simulink model "Final_System_Model_V2"  (R2018a)
settings: Solver=VariableStepAuto  StartTime=0  StopTime=inf  RelTol=1e-3
PreLoadFcn:
  | Ts_Power=1e-6;
  | Ts_Control=100e-6;
undefined symbols (not defined in the file): DiscIntNeverNeededParam, FC, FuelCellLoadFcn, gcbh, Ion, Lithium, sigbuilder_block, sps_rtmsupport
libraries: powerlib x20, simulink x10, fl_lib x8, nesl_utility x6, powerlib_meascontrol x5, electricdrivelib x1, spsFuelCellModel x1, re_lib x1
(part 4 of 4)

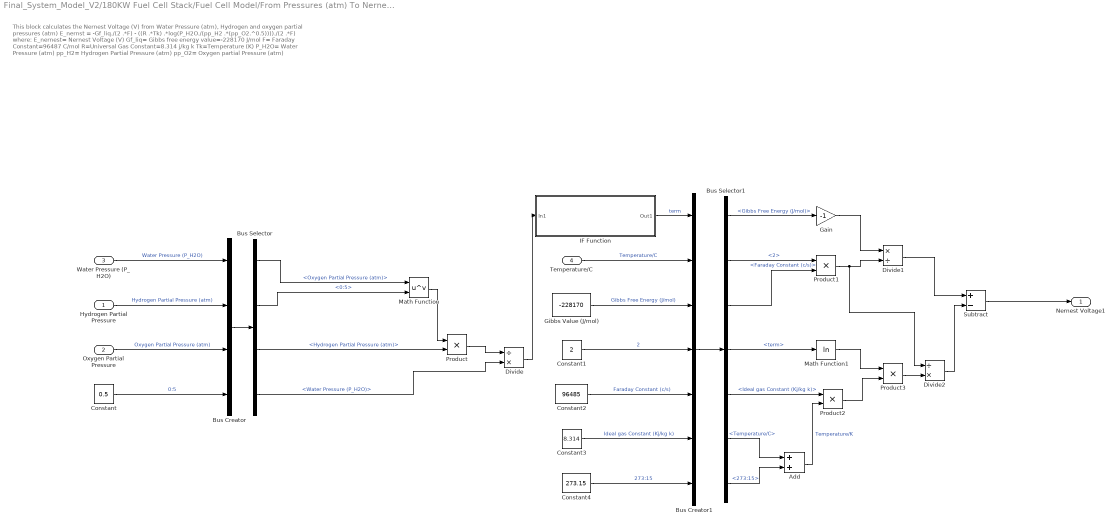
== system Final_System_Model_V2/180KW Fuel Cell Stack/Fuel Cell Model/From Pressures (atm) To Nernest Voltage (V)/From Partial Pressures (atm) To Nernest Voltage (V) ==
  note: This block calculates the Nernest Voltage (V) from Water Pressure (atm), Hydrogen and oxygen partial pressures (atm)
      | E_nernst = -Gf_liq./(2 .*F) - ((R .*Tk) .*log(P_H2O./(pp_H2 .*(pp_O2.^0.5))))./(2 .*F)
      | where: E_nernest= Nernest Voltage (V)
      | Gf_liq= Gibbs free energy value=-228170 J/mol
      | F= Faraday Constant=96487 C/mol
      | R=Universal Gas Constant=8.314 j/kg k
      | Tk=Temperature (K)
      | P_H2O= Water Pressure (atm)
      | pp_H2= Hydrogen Partial Pressure (atm)
      | pp_O2= Oxygen partial Pressure (atm)
  Hydrogen Partial Pressure : Inport
  Oxygen Partial Pressure : Inport  Port=2
  Water Pressure (P_H2O) : Inport  Port=3
  Temperature/C : Inport  Port=4
  Add : Sum
  Bus Creator : BusCreator  Inputs=4
  Bus Creator1 : BusCreator  Inputs=7
  Bus Selector : BusSelector  OutputSignals=Oxygen Partial Pressure (atm),0:5,Hydrogen Partial Pressure (atm),Water Pressure (P_H2O)
  Bus Selector1 : BusSelector  OutputSignals=Gibbs Free Energy (J/mol),2,Faraday Constant (c/s),term,Ideal gas Constant (Kj/kg k),Temperature/C,273:15
  Constant : Constant  Value=0.5
  Constant1 : Constant  Value=2
  Constant2 : Constant  Value=96485
  Constant3 : Constant  Value=8.314
  Constant4 : Constant  Value=273.15
  Divide : Product  Inputs=/*
  Divide1 : Product  Inputs=*/
  Divide2 : Product  Inputs=/*
  Gain : Gain  Gain=-1
  Gibbs Value (J/mol) : Constant  Value=-228170
  IF Function : Subsystem
  Math Function : Math  Operator=pow  SaturateOnIntegerOverflow=on
  Math Function1 : Math  Operator=log  SaturateOnIntegerOverflow=on
  Product{,1..3} (4 alike) : Product
  Subtract : Sum  Inputs=+-
  Nernest Voltage1 : Outport
  wires:
  Gibbs Value (J/mol)/1 -> Bus Creator1/3  "Gibbs Free Energy (J/mol)"
  Oxygen Partial Pressure/1 -> Bus Creator/3  "Oxygen Partial Pressure (atm)"
  Water Pressure (P_H2O)/1 -> Bus Creator/1  "Water Pressure (P_H2O)"
  Hydrogen Partial Pressure/1 -> Bus Creator/2  "Hydrogen Partial Pressure (atm)"
  Temperature/C/1 -> Bus Creator1/2  "Temperature/C"
  Bus Creator/1 -> Bus Selector/1
  Bus Selector/2 -> Math Function/2  "<0:5>"
  Constant/1 -> Bus Creator/4  "0:5"
  Bus Selector/1 -> Math Function/1  "<Oxygen Partial Pressure (atm)>"
  Bus Selector/3 -> Product/2  "<Hydrogen Partial Pressure (atm)>"
  Math Function/1 -> Product/1
  Bus Selector/4 -> Divide/2  "<Water Pressure (P_H2O)>"
  Product/1 -> Divide/1
  Divide/1 -> IF Function/1(In1)
  IF Function/1(Out1) -> Bus Creator1/1  "term"
  Bus Creator1/1 -> Bus Selector1/1
  Constant1/1 -> Bus Creator1/4  "2"
  Constant2/1 -> Bus Creator1/5  "Faraday Constant (c/s)"
  Bus Selector1/1 -> Gain/1  "<Gibbs Free Energy (J/mol)>"
  Gain/1 -> Divide1/1
  Bus Selector1/2 -> Product1/1  "<2>"
  Bus Selector1/3 -> Product1/2  "<Faraday Constant (c/s)>"
  Product1/1 -> Divide2/1, Divide1/2
  Divide1/1 -> Subtract/1
  Bus Selector1/4 -> Math Function1/1  "<term>"
  Math Function1/1 -> Product3/1
  Constant3/1 -> Bus Creator1/6  "Ideal gas Constant (Kj/kg k)"
  Constant4/1 -> Bus Creator1/7  "273:15"
  Bus Selector1/5 -> Product2/1  "<Ideal gas Constant (Kj/kg k)>"
  Bus Selector1/6 -> Add/1  "<Temperature/C>"
  Bus Selector1/7 -> Add/2  "<273:15>"
  Add/1 -> Product2/2  "Temperature/K"
  Product2/1 -> Product3/2
  Product3/1 -> Divide2/2
  Divide2/1 -> Subtract/2
  Subtract/1 -> Nernest Voltage1/1

== system Final_System_Model_V2/Electrolyzer Stack/electrolyser stack/electrolyser cell/(1//T)//(1//T_ref) ==
  In1 : Inport
  In2 : Inport  Port=2
  Constant : Constant
  Divide1 : Product  Inputs=*/
  Divide2 : Product  Inputs=*/
  Out1 : Outport
  wires:
  Divide1/1 -> Divide2/1
  Constant/1 -> Divide1/1
  In2/1 -> Divide2/2
  Divide2/1 -> Out1/1
  In1/1 -> Divide1/2

== system Final_System_Model_V2/Electrolyzer Stack/electrolyser stack/electrolyser cell/Eta_B ==
  In1 : Inport
  In2 : Inport  Port=2
  In3 : Inport  Port=3
  In4 : Inport  Port=4
  L_B : Constant  Value=175e-4
  Product : Product  Inputs=*/
  Product1 : Product
  segma_B : Subsystem
  Out1 : Outport
  wires:
  segma_B/1(Out1) -> Product/2
  L_B/1 -> Product/1
  Product1/1 -> Out1/1
  In3/1 -> Product1/2
  Product/1 -> Product1/1
  In2/1 -> segma_B/2(In2)
  In4/1 -> segma_B/3(In4)
  In1/1 -> segma_B/1(In1)

== system Final_System_Model_V2/Electrolyzer Stack/electrolyser stack/electrolyser cell/H2 flow rate ==
  In1 : Inport
  In2 : Inport  Port=2
  In3 : Inport  Port=3
  Divide : Product  Inputs=*/
  Multiply : Product
  Out1 : Outport
  wires:
  Multiply/1 -> Divide/1
  In1/1 -> Multiply/1
  In3/1 -> Multiply/2
  In2/1 -> Divide/2
  Divide/1 -> Out1/1

== system Final_System_Model_V2/Electrolyzer Stack/electrolyser stack/electrolyser cell/V_0 ==
  In1 : Inport
  Add : Sum  Inputs=+-
  Add1 : Sum  Inputs=+-
  Constant : Constant  Value=8.46e-4
  OCV : Constant  Value=1.229
  Product : Product
  T_ref : Constant  Value=298
  Out1 : Outport
  wires:
  OCV/1 -> Add/1
  Add/1 -> Out1/1
  Product/1 -> Add/2
  T_ref/1 -> Add1/2
  In1/1 -> Add1/1
  Constant/1 -> Product/1
  Add1/1 -> Product/2

== system Final_System_Model_V2/Electrolyzer Stack/electrolyser stack/electrolyser cell/eta_a ==
  In1 : Inport
  In2 : Inport  Port=2
  In3 : Inport  Port=3
  In4 : Inport  Port=4
  In5 : Inport  Port=5
  In6 : Inport  Port=6
  B_a : Constant  Value=5
  Divide : Product  Inputs=*/
  Divide1 : Product  Inputs=*/
  Gain : Gain  Gain=0.5
  Multiply : Product
  Multiply1 : Product  Inputs=3
  Multiply2 : Product
  Sin : Trigonometry  Operator=asinh
  m_a : Subsystem
  n_a : Subsystem
  v_a : Constant  Value=3
  Out1 : Outport
  wires:
  n_a/1(Out1) -> Divide1/1
  B_a/1 -> Multiply1/1
  Divide1/1 -> Gain/1
  In1/1 -> n_a/1(In1)
  Sin/1 -> Multiply2/1
  Multiply/1 -> Divide/1
  In6/1 -> Multiply1/3
  Gain/1 -> Sin/1
  Multiply1/1 -> Divide/2
  In3/1 -> n_a/3(In3), m_a/1(In1)
  Multiply2/1 -> Out1/1
  Divide/1 -> Multiply2/2
  v_a/1 -> Multiply1/2
  m_a/1(Out1) -> Divide1/2
  In5/1 -> Multiply/2
  In4/1 -> Multiply/1
  In2/1 -> n_a/2(In2)

== system Final_System_Model_V2/Electrolyzer Stack/electrolyser stack/electrolyser cell/eta_c ==
  In1 : Inport
  In2 : Inport  Port=2
  In3 : Inport  Port=3
  In4 : Inport  Port=4
  In5 : Inport  Port=5
  B_c : Constant  Value=5
  Divide : Product  Inputs=*/
  Divide1 : Product  Inputs=*/
  Gain : Gain  Gain=0.5
  Multiply : Product
  Multiply1 : Product  Inputs=3
  Multiply2 : Product
  Sin : Trigonometry  Operator=asinh
  m_c : Subsystem
  n_c : Subsystem
  v_c : Constant  Value=-1
  Out1 : Outport
  wires:
  In1/1 -> n_c/1(In1)
  In2/1 -> Multiply/1, n_c/2(In2)
  Multiply/1 -> Divide/1
  Divide1/1 -> Gain/1
  n_c/1(Out1) -> Divide1/1
  v_c/1 -> Multiply1/3
  In4/1 -> m_c/1(In1), n_c/3(In3)
  B_c/1 -> Multiply1/1
  Multiply1/1 -> Divide/2
  Sin/1 -> Multiply2/1
  m_c/1(Out1) -> Divide1/2
  Divide/1 -> Multiply2/2
  Gain/1 -> Sin/1
  Multiply2/1 -> Out1/1
  In3/1 -> Multiply/2
  In5/1 -> Multiply1/2

== system Final_System_Model_V2/Solar Panel + Solar Charge Controller/PV Insert inputs here/Subsystem/C to K Converter  ==
  T_o : Inport
  Sum : Sum  Inputs=|++
  Sum1 : Sum  Inputs=|++
  T_ref : Constant  Value=25
  constant : Constant  Value=273.12
  T_ak : Outport
  T_rk : Outport  Port=2
  wires:
  constant/1 -> Sum1/1, Sum/2
  T_o/1 -> Sum/1  "T_act (c)"
  T_ref/1 -> Sum1/2  "T_ref (c)"
  Sum/1 -> T_ak/1  "T_act(k)"
  Sum1/1 -> T_rk/1  "T_ref(k)"

== system Final_System_Model_V2/Solar Panel + Solar Charge Controller/PV Insert inputs here/Subsystem/I o ==
  T_ak : Inport
  T_rk : Inport  Port=2
  I_on : Inport  Port=3
  Constant : Constant
  Electron charge : Constant  Value=1.6*10^(-19)
  Exp(fn(1)) : Fcn  Expr=exp(u(1))
  Fcn : Fcn  Expr=(u(1))^3
  Product : Product  Inputs=/***/
  Product1 : Product  Inputs=*/
  Product2 : Product  Inputs=*/
  Product3 : Product  Inputs=*/
  Product4 : Product  Inputs=3
  Sum : Sum  Inputs=|+-
  band gap energy (Eg) : Constant  Value=1.1
  boltzamann constant : Constant  Value=1.3805*10^(-23)
  ideality factor depend on material : Constant  Value=1.14
  I_o : Outport
  wires:
  Electron charge/1 -> Product/2  "e"
  boltzamann constant/1 -> Product/1  "k"
  Product2/1 -> Sum/2  "1/T"
  I_on/1 -> Product4/3  "I_on"
  band gap energy (Eg)/1 -> Product/3  "Eg"
  Sum/1 -> Product/4  "((1/Tn)-(1/T))"
  Product3/1 -> Fcn/1  "T/Tn"
  Product1/1 -> Sum/1  "1/Tn"
  Constant/1 -> Product2/1, Product1/1
  ideality factor depend on material/1 -> Product/5  "a"
  T_ak/1 -> Product3/1, Product2/2
  Fcn/1 -> Product4/2  "(T/Tn)^3"
  Product/1 -> Exp(fn(1))/1  "Fn(1)"
  Exp(fn(1))/1 -> Product4/1  "Exp(fn(1))"
  T_rk/1 -> Product1/2, Product3/2
  Product4/1 -> I_o/1

== system Final_System_Model_V2/Solar Panel + Solar Charge Controller/PV Insert inputs here/Subsystem/I on ==
  T_ref : Inport
  I_scn : Inport  Port=2
  Num series : Inport  Port=3
  V_oc : Inport  Port=4
  Electron charge : Constant  Value=1.6*10^(-19)
  Fcn : Fcn  Expr=(u(1))/(exp(u(2))-u(1))
  Mux : Mux  Inputs=3
  Product : Product  Inputs=//**//
  boltzamann constant : Constant  Value=1.3805*10^(-23)
  constant : Constant
  ideality factor : Constant  Value=1.1415
  I_on : Outport
  wires:
  Num series/1 -> Product/1  "num_series_cells"
  boltzamann constant/1 -> Product/2  "K"
  Electron charge/1 -> Product/3  "q"
  ideality factor/1 -> Product/5  "a"
  T_ref/1 -> Product/6  "T_ref(k)"
  Product/1 -> Mux/2
  I_scn/1 -> Mux/1
  constant/1 -> Mux/3
  Mux/1 -> Fcn/1
  Fcn/1 -> I_on/1
  V_oc/1 -> Product/4

== system Final_System_Model_V2/Solar Panel + Solar Charge Controller/PV Insert inputs here/Subsystem/I ph due to radiation  ==
  insolation : Inport
  T_ak : Inport  Port=2
  T_rk : Inport  Port=3
  I_scn : Inport  Port=4
  Product : Product
  Product1 : Product
  SC_temp COFF const : Constant  Value=0.0017
  Sum : Sum  Inputs=|++
  Sum1 : Sum  Inputs=|+-
  I_photon : Outport
  wires:
  Product/1 -> I_photon/1  "photons current"
  insolation/1 -> Product/1
  T_ak/1 -> Sum1/1  "actual temp(k)"
  T_rk/1 -> Sum1/2  "referance temp(k)"
  Sum/1 -> Product/2
  I_scn/1 -> Sum/2  "nominal short circuit current"
  Product1/1 -> Sum/1
  SC_temp COFF const/1 -> Product1/1
  Sum1/1 -> Product1/2

== system Final_System_Model_V2/Solar Panel + Solar Charge Controller/PV Insert inputs here/Subsystem/I pv ==
  V_PV : Inport
  I_photon : Inport  Port=2
  I_o : Inport  Port=3
  Ns*A*Kt1 : Inport  Port=4
  Rp Shunt resistance : Inport  Port=5
  Electron charge : Constant  Value=1.6*10^(-19)
  IPV = u(3)-u(4)*(exp((u(2)*(u(1)+u(6)))/(u(5)))-1) : Fcn  Expr=u(3)-u(4)*(exp((u(2)*(u(1)+u(6)))/(u(5)))-1)-u(7)
  Mux : Mux  Inputs=7
  Product : Product  Inputs=*/
  Rs : Gain  Gain=.4
  Sum : Sum  Inputs=|++
  I_PV : Outport
  wires:
  IPV = u(3)-u(4)*(exp((u(2)*(u(1)+u(6)))/(u(5)))-1)/1 -> I_PV/1, Rs/1  "I_PV"
  Ns*A*Kt1/1 -> Mux/5
  Mux/1 -> IPV = u(3)-u(4)*(exp((u(2)*(u(1)+u(6)))/(u(5)))-1)/1
  I_o/1 -> Mux/4  "I_o"
  Rs/1 -> Sum/2, Mux/6  "I_PV*Rs"
  Electron charge/1 -> Mux/2  "q"
  I_photon/1 -> Mux/3  "I_ph"
  V_PV/1 -> Sum/1, Mux/1  "V_PV"
  Sum/1 -> Product/1
  Rp Shunt resistance/1 -> Product/2  "Shunt resistance"
  Product/1 -> Mux/7

== system Final_System_Model_V2/Solar Panel + Solar Charge Controller/PV Insert inputs here/Subsystem/NsAKt Thermal voltafe ==
  T_ak T in kelven : Inport
  N_series series cells : Constant  Value=96
  Product4 : Product  Inputs=4
  boltzamann constant : Constant  Value=1.3805*10^(-23)
  ideality factor depend on material : Constant  Value=1.17
  Ns*a*Kt : Outport
  wires:
  Product4/1 -> Ns*a*Kt/1
  boltzamann constant/1 -> Product4/2
  ideality factor depend on material/1 -> Product4/3
  T_ak T in kelven/1 -> Product4/1
  N_series series cells/1 -> Product4/4

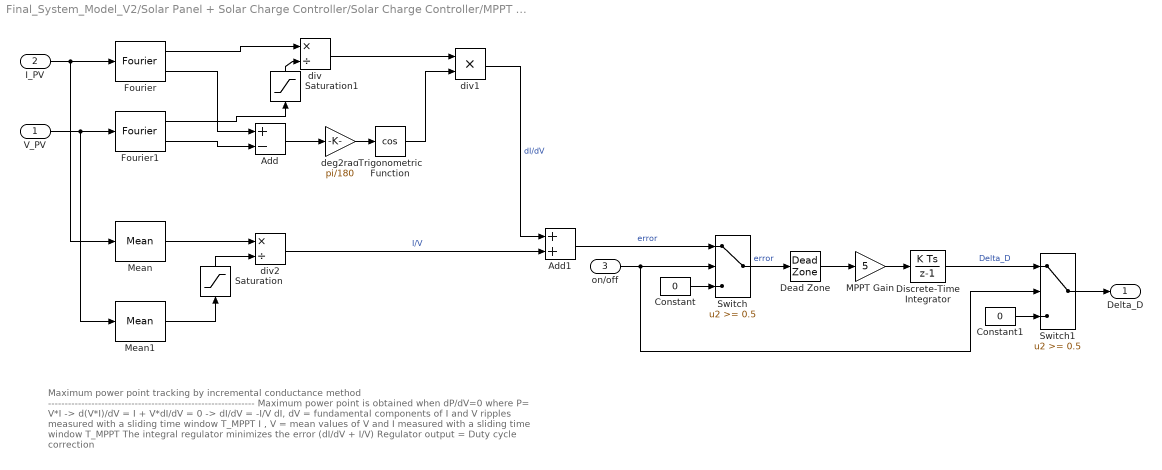
== system Final_System_Model_V2/Solar Panel + Solar Charge Controller/Solar Charge Controller/MPPT Controller using  "Incremental Conductance + Integral Regulator "  technique /MPPT ==
  note: Maximum power point tracking by incremental conductance method
      | --------------------------------------------------------------
      | Maximum power point is obtained when dP/dV=0  where P= V*I
      | -> d(V*I)/dV = I + V*dI/dV = 0
      | -> dI/dV = -I/V
      |
      | dI, dV  = fundamental components of I and V ripples measured with a sliding time window T_MPPT
      | I , V   = mean values of V and I measured with a sliding time window T_MPPT
      |
      | The integral regulator minimizes the error (dI/dV + I/V)
      | Regulator output = Duty cycle correction
  V_PV : Inport
  I_PV : Inport  Port=2
  on/off : Inport  Port=3
  Add : Sum  Inputs=+-
  Add1 : Sum
  Constant : Constant  Value=0
  Constant1 : Constant  Value=0
  Dead Zone : DeadZone  LowerValue=-0.05  UpperValue=0.05  SaturateOnIntegerOverflow=on
  Discrete-Time Integrator : DiscreteIntegrator  SampleTime=Ts_Control  LimitOutput=on  UpperSaturationLimit=1  LowerSaturationLimit=-1  ICPrevOutput=DiscIntNeverNeededParam  ICPrevScaledInput=DiscIntNeverNeededParam
  Fourier : powerlib_meascontrol/Measurements/Fourier  Freq=1/T_MPPT  n=1  InInit=[0, 0]  Ts=Ts_Control
      settings: SourceProductName=Simscape Power Systems
  Fourier1 : powerlib_meascontrol/Measurements/Fourier  Freq=1/T_MPPT  n=1  InInit=[0, 0]  Ts=Ts_Control
      settings: SourceProductName=Simscape Power Systems
  MPPT Gain : Gain  Gain=5
  Mean : powerlib_meascontrol/Measurements/Mean  Freq=1/T_MPPT  Vinit=0  Ts=Ts_Control
  Mean1 : powerlib_meascontrol/Measurements/Mean  Freq=1/T_MPPT  Vinit=0  Ts=Ts_Control
  Saturation : Saturate  UpperLimit=inf  LowerLimit=eps
  Saturation1 : Saturate  UpperLimit=inf  LowerLimit=eps
  Switch : Switch  Threshold=0.5
  Switch1 : Switch  Threshold=0.5
  Trigonometric Function : Trigonometry  Operator=cos
  deg2rad : Gain  Gain=pi/180
  div : Product  Inputs=*/  RndMeth=Zero
  div1 : Product  Inputs=**  RndMeth=Zero
  div2 : Product  Inputs=*/  RndMeth=Zero
  Delta_D : Outport
  wires:
  Dead Zone/1 -> MPPT Gain/1
  Switch/1 -> Dead Zone/1  "error"
  Saturation1/1 -> div/2
  Saturation/1 -> div2/2
  Switch1/1 -> Delta_D/1
  on/off/1 -> Switch/2, Switch1/2
  Constant1/1 -> Switch1/3
  Discrete-Time Integrator/1 -> Switch1/1  "Delta_D"
  Constant/1 -> Switch/3
  MPPT Gain/1 -> Discrete-Time Integrator/1
  Add1/1 -> Switch/1  "error"
  div2/1 -> Add1/2  "I/V"
  Mean1/1 -> Saturation/1
  Mean/1 -> div2/1
  div1/1 -> Add1/1  "dI/dV"
  Trigonometric Function/1 -> div1/2
  div/1 -> div1/1
  deg2rad/1 -> Trigonometric Function/1
  Add/1 -> deg2rad/1
  Fourier1/1 -> Saturation1/1
  Fourier1/2 -> Add/2
  Fourier/2 -> Add/1
  V_PV/1 -> Mean1/1, Fourier1/1
  I_PV/1 -> Mean/1, Fourier/1
  Fourier/1 -> div/1

== system Final_System_Model_V2/Solar Panel + Solar Charge Controller/Solar Charge Controller MPPT it is a device which track a point which has the max power/MPPT /P&O  ==
  I_pv : Inport
  V_PV : Inport  Port=2
  P & O : Subsystem
  Saturation : Saturate  UpperLimit=1
  Subsystem1 : Subsystem
  Signal : Outport
  wires:
  P & O/1(signal) -> Saturation/1
  V_PV/1 -> P & O/2(Vpv)
  Saturation/1 -> Subsystem1/1(In1)
  Subsystem1/1(Out1) -> Signal/1
  I_pv/1 -> P & O/1(Ipv)

== system Final_System_Model_V2/180KW Fuel Cell Stack/Fuel Cell Model/ From Current Density (A//cm^2) To Overvoltages (V)/Concentration Overvoltage/IF Function ==
  In1 : Inport
  Compare To Zero : simulink/Logic and Bit Operations/Compare To Zero  relop=<=  OutDataTypeStr=boolean
  If : If  IfExpression=u1 == 0
  If Action Subsystem : Subsystem  TreatAsAtomicUnit=on
  If Action Subsystem1 : Subsystem  TreatAsAtomicUnit=on
  Merge : Merge  InitialOutput=1
  Out1 : Outport
  wires:
  If Action Subsystem1/1(Out1) -> Merge/2
  Compare To Zero/1 -> If/1
  Merge/1 -> Out1/1
  In1/1 -> If Action Subsystem/1(In1), Compare To Zero/1
  If/2 -> If Action Subsystem1/Action
  If Action Subsystem/1(Out1) -> Merge/1
  If/1 -> If Action Subsystem/Action

== system Final_System_Model_V2/180KW Fuel Cell Stack/Fuel Cell Model/From Pressures (atm) To Nernest Voltage (V)/From Absolute Pressure (atm) To Partial Pressures (atm)/Hydrogen Partial Pressure Output ==
  note: This block calculates the Hydrogen partial Pressure (pp_H2)(atm)
      | pp_H2 = 0.5 .*((P_H2)./(exp(1.653 .*i./(Tk.^1.334))))-P_H2O
      | where: pp_H2= Hydrogen Partial Pressure (atm)
      | i=Current Density (A/cm^2)
      | Tk= Temperature in Kelvin
      | P_H2O= Water pressure (atm)
  Hydrogen Pressure (P_H2) : Inport
  Temperature/C : Inport  Port=2
  Current Density (i ) : Inport  Port=3
  Water Pressure : Inport  Port=4
  Add : Sum
  Bus Creator : BusCreator  Inputs=6
  Bus Selector : BusSelector  OutputSignals=Stack Temperature (C),273:15,1:653,Current Density (A/cm^2),Hydrogen Pressure (atm),Water Pressure(atm)
  Constant : Constant  Value=273.15
  Constant1 : Constant  Value=1.653
  Constant2 : Constant  Value=1.334
  Divide : Product  Inputs=/*
  Divide1 : Product  Inputs=/*
  Gain : Gain  Gain=0.5
  Math Function : Math  Operator=pow  SaturateOnIntegerOverflow=on
  Math Function1 : Math  SaturateOnIntegerOverflow=on
  Product : Product
  Subtract : Sum  Inputs=+-
  Hydrogen Partial Pressure (pp_H2) : Outport
  wires:
  Water Pressure/1 -> Bus Creator/4
  Temperature/C/1 -> Bus Creator/3
  Current Density (i )/1 -> Bus Creator/2
  Hydrogen Pressure (P_H2)/1 -> Bus Creator/1
  Bus Creator/1 -> Bus Selector/1
  Bus Selector/5 -> Divide1/2  "<Hydrogen Pressure (atm)>"
  Bus Selector/1 -> Add/1  "<Stack Temperature (C)>"
  Constant/1 -> Bus Creator/5  "273:15"
  Add/1 -> Math Function/1  "Temperature/K"
  Constant1/1 -> Bus Creator/6  "1:653"
  Bus Selector/2 -> Add/2  "<273:15>"
  Bus Selector/3 -> Product/1  "<1:653>"
  Bus Selector/4 -> Product/2  "<Current Density (A/cm^2)>"
  Product/1 -> Divide/2
  Divide/1 -> Math Function1/1
  Constant2/1 -> Math Function/2
  Math Function/1 -> Divide/1
  Math Function1/1 -> Divide1/1
  Divide1/1 -> Gain/1
  Bus Selector/6 -> Subtract/2  "<Water Pressure(atm)>"
  Subtract/1 -> Hydrogen Partial Pressure (pp_H2)/1
  Gain/1 -> Subtract/1

== system Final_System_Model_V2/180KW Fuel Cell Stack/Fuel Cell Model/From Pressures (atm) To Nernest Voltage (V)/From Absolute Pressure (atm) To Partial Pressures (atm)/Oxygen Partial Pressure Output ==
  note: This block calculates the Oxygen Partial Pressure (atm)
      | pp_O2 = (P_air./exp(4.192 .*i/(Tk.^1.334)))-P_H2O
      |
      | where: pp_O2= Oxygen Partial Pressure (atm)
      | P_air= Air Pressure (atm)
      | i= Current Density (A/cm^2)
      | Tk= Temperature (K)
      | P_H2O=Water Pressure (atm)
  Air Pressure (P_air) : Inport
  Temperature/C : Inport  Port=2
  Current Density/i : Inport  Port=3
  Water Pressure : Inport  Port=4
  Add : Sum
  Bus Creator : BusCreator  Inputs=7
  Bus Selector : BusSelector  OutputSignals=Stack Temperature (C),273:15,1:334,Current Density (A/cm^2),4:192,Air Pressure (atm),Water Pressure(atm)
  Constant : Constant  Value=273.15
  Constant1 : Constant  Value=4.192
  Constant2 : Constant  Value=1.334
  Divide : Product  Inputs=/*
  Divide1 : Product  Inputs=/*
  Math Function : Math  Operator=pow  SaturateOnIntegerOverflow=on
  Math Function1 : Math  SaturateOnIntegerOverflow=on
  Product : Product
  Subtract : Sum  Inputs=+-
  Oxygen Partial Pressure pp_O2 : Outport
  wires:
  Current Density/i/1 -> Bus Creator/2
  Water Pressure/1 -> Bus Creator/4
  Temperature/C/1 -> Bus Creator/3
  Air Pressure (P_air)/1 -> Bus Creator/1
  Constant/1 -> Bus Creator/5  "273:15"
  Constant1/1 -> Bus Creator/6  "4:192"
  Constant2/1 -> Bus Creator/7  "1:334"
  Bus Creator/1 -> Bus Selector/1
  Bus Selector/1 -> Add/1  "<Stack Temperature (C)>"
  Bus Selector/2 -> Add/2  "<273:15>"
  Add/1 -> Math Function/1  "Temperature/K"
  Bus Selector/3 -> Math Function/2  "<1:334>"
  Bus Selector/4 -> Product/1  "<Current Density (A/cm^2)>"
  Bus Selector/5 -> Product/2  "<4:192>"
  Product/1 -> Divide/2
  Math Function/1 -> Divide/1
  Divide/1 -> Math Function1/1
  Math Function1/1 -> Divide1/1
  Bus Selector/6 -> Divide1/2  "<Air Pressure (atm)>"
  Divide1/1 -> Subtract/1
  Bus Selector/7 -> Subtract/2  "<Water Pressure(atm)>"
  Subtract/1 -> Oxygen Partial Pressure pp_O2/1  "Oxygen Partial Pressure pp_O2 (atm)"

== system Final_System_Model_V2/180KW Fuel Cell Stack/Fuel Cell Model/From Pressures (atm) To Nernest Voltage (V)/From Absolute Pressure (atm) To Partial Pressures (atm)/Water Pressure output ==
  note: This block calculates the water saturation Pressure (atm) from the Fuel Cell Temperature (k)
      | x = -2.1794 + 0.02953 .*Tc-9.1837 .*(10.^-5) .*(Tc.^2) + 1.4454 .*(10.^-7) .*(Tc.^3);
      | where: x=Water Saturation Pressure (atm)
      | Tc= Temperature in degree celsius
  Temperature/C : Inport
  -1 : Constant  Value=-7
  -2 : Constant  Value=3
  -5 : Constant  Value=-5
  0.02953 : Constant  Value=0.02953
  0.1 : Constant  Value=9.1837
  0.2 : Constant  Value=1.4454
  Add : Sum  Inputs=+++-
  Constant4 : Constant  Value=-2.1794
  Math Function4 : Math  Operator=10^u  SaturateOnIntegerOverflow=on
  Math Function5 : Math  Operator=square  SaturateOnIntegerOverflow=on
  Math Function6 : Math  Operator=10^u  SaturateOnIntegerOverflow=on
  Math Function7 : Math  Operator=pow  SaturateOnIntegerOverflow=on
  Product1 : Product  Inputs=3
  Product2 : Product
  Product3 : Product  Inputs=3
  "water  pressure " : Math  Operator=10^u  SaturateOnIntegerOverflow=on
  Water Pressure : Outport
  wires:
  Add/1 -> "water  pressure "/1
  0.2/1 -> Product3/1
  Math Function7/1 -> Product3/3
  "water  pressure "/1 -> Water Pressure/1  "Water Pressure(atm)"
  0.02953/1 -> Product2/1
  0.1/1 -> Product1/1
  -5/1 -> Math Function4/1
  Math Function4/1 -> Product1/2
  -1/1 -> Math Function6/1
  Temperature/C/1 -> Product2/2, Math Function5/1, Math Function7/1
  Math Function5/1 -> Product1/3
  -2/1 -> Math Function7/2
  Product2/1 -> Add/2
  Product3/1 -> Add/3
  Math Function6/1 -> Product3/2
  Constant4/1 -> Add/1
  Product1/1 -> Add/4

== system Final_System_Model_V2/180KW Fuel Cell Stack/Fuel Cell Model/From Pressures (atm) To Nernest Voltage (V)/From Partial Pressures (atm) To Nernest Voltage (V)/IF Function ==
  In1 : Inport
  Constant1 : Constant
  If : If
  If Action Subsystem : Subsystem  TreatAsAtomicUnit=on
  If Action Subsystem1 : Subsystem  TreatAsAtomicUnit=on
  Merge : Merge
  Out1 : Outport
  wires:
  Constant1/1 -> If Action Subsystem1/1(In1)
  If Action Subsystem1/1(Out1) -> Merge/2
  If/1 -> If Action Subsystem/Action
  If/2 -> If Action Subsystem1/Action
  In1/1 -> If Action Subsystem/1(In1), If/1
  Merge/1 -> Out1/1
  If Action Subsystem/1(Out1) -> Merge/1

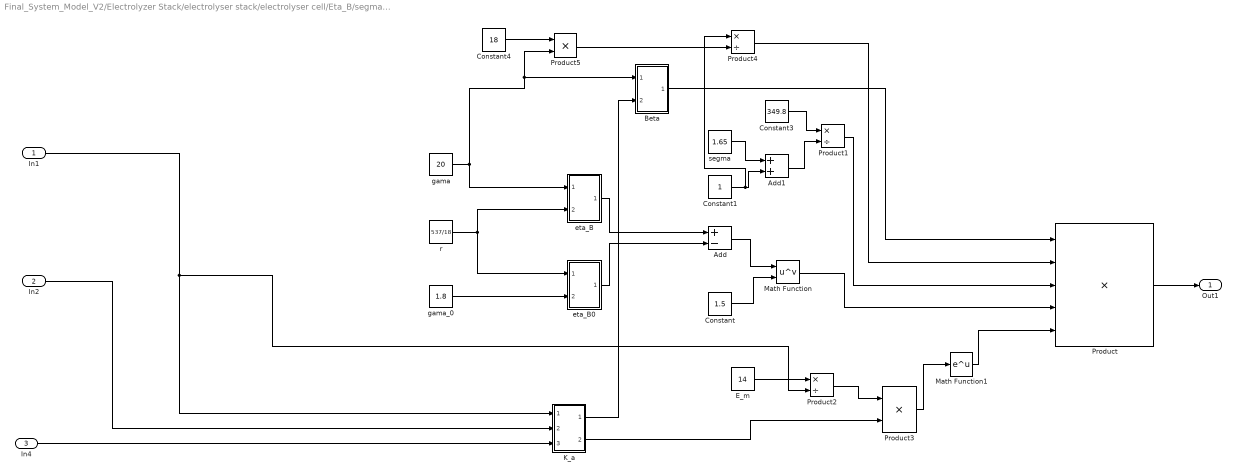
== system Final_System_Model_V2/Electrolyzer Stack/electrolyser stack/electrolyser cell/Eta_B/segma_B ==
  In1 : Inport
  In2 : Inport  Port=2
  In4 : Inport  Port=3
  Add : Sum  Inputs=+-
  Add1 : Sum
  Beta : Subsystem
  Constant : Constant  Value=1.5
  Constant1 : Constant
  Constant3 : Constant  Value=349.8
  Constant4 : Constant  Value=18
  E_m : Constant  Value=14
  K_a : Subsystem
  Math Function : Math  Operator=pow  SaturateOnIntegerOverflow=on
  Math Function1 : Math  SaturateOnIntegerOverflow=on
  Product : Product  Inputs=5
  Product1 : Product  Inputs=*/
  Product2 : Product  Inputs=*/
  Product3 : Product
  Product4 : Product  Inputs=*/
  Product5 : Product  Inputs=**
  eta_B : Subsystem
  eta_B0 : Subsystem
  gama : Constant  Value=20
  gama_0 : Constant  Value=1.8
  r : Constant  Value=537/18
  segma : Constant  Value=1.65
  Out1 : Outport
  wires:
  Constant1/1 -> Product4/1, Add1/2
  Math Function1/1 -> Product/5
  eta_B0/1(Out1) -> Add/2
  In4/1 -> K_a/3(In3)
  In1/1 -> Product2/2, K_a/1(In1)
  In2/1 -> K_a/2(In2)
  Product5/1 -> Product4/2
  K_a/1(Out1) -> Beta/2(In2)
  Constant3/1 -> Product1/1
  Math Function/1 -> Product/4
  E_m/1 -> Product2/1
  Constant/1 -> Math Function/2
  Add1/1 -> Product1/2
  segma/1 -> Add1/1
  Product1/1 -> Product/3
  gama_0/1 -> eta_B0/2(In2)
  Product3/1 -> Math Function1/1
  Add/1 -> Math Function/1
  Beta/1(Out1) -> Product/1
  Constant4/1 -> Product5/1
  Product4/1 -> Product/2
  gama/1 -> Product5/2, Beta/1(In1), eta_B/1(In1)
  r/1 -> eta_B0/1(In1), eta_B/2(In2)
  Product/1 -> Out1/1
  eta_B/1(Out1) -> Add/1
  K_a/2(Out2) -> Product3/2
  Product2/1 -> Product3/1

== system Final_System_Model_V2/Electrolyzer Stack/electrolyser stack/electrolyser cell/eta_a/m_a ==
  In1 : Inport
  Constant : Constant
  Divide : Product  Inputs=*/
  Subtract : Sum  Inputs=+-
  limiting current : Constant  Value=2
  Out1 : Outport
  wires:
  In1/1 -> Divide/1
  limiting current/1 -> Divide/2
  Constant/1 -> Subtract/1
  Subtract/1 -> Out1/1
  Divide/1 -> Subtract/2

== system Final_System_Model_V2/Electrolyzer Stack/electrolyser stack/electrolyser cell/eta_a/n_a ==
  In1 : Inport
  In2 : Inport  Port=2
  In3 : Inport  Port=3
  Divide : Product  Inputs=*/
  i_a0 : Subsystem
  Out1 : Outport
  wires:
  In2/1 -> i_a0/1(In1)
  i_a0/1(Out1) -> Divide/2
  Divide/1 -> Out1/1
  In1/1 -> i_a0/2(In2)
  In3/1 -> Divide/1

== system Final_System_Model_V2/Electrolyzer Stack/electrolyser stack/electrolyser cell/eta_c/m_c ==
  In1 : Inport
  Constant : Constant
  Divide : Product  Inputs=*/
  Subtract : Sum  Inputs=+-
  limiting current : Constant  Value=0.00023
  Out1 : Outport
  wires:
  Constant/1 -> Subtract/1
  Subtract/1 -> Out1/1
  limiting current/1 -> Divide/2
  Divide/1 -> Subtract/2
  In1/1 -> Divide/1

== system Final_System_Model_V2/Electrolyzer Stack/electrolyser stack/electrolyser cell/eta_c/n_c ==
  In1 : Inport
  In2 : Inport  Port=2
  In3 : Inport  Port=3
  Divide : Product  Inputs=*/
  i_c0 : Subsystem
  Out1 : Outport
  wires:
  In2/1 -> i_c0/1(In1)
  i_c0/1(Out1) -> Divide/2
  In1/1 -> i_c0/2(In2)
  Divide/1 -> Out1/1
  In3/1 -> Divide/1

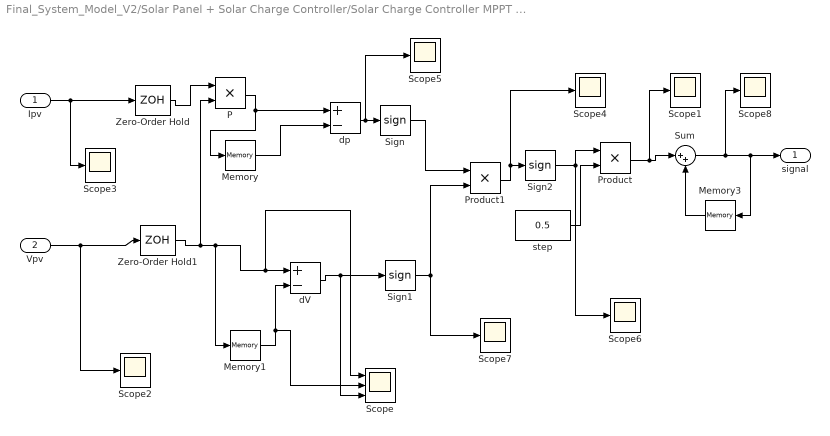
== system Final_System_Model_V2/Solar Panel + Solar Charge Controller/Solar Charge Controller MPPT it is a device which track a point which has the max power/MPPT /P&O /P & O ==
  Ipv : Inport
  Vpv : Inport  Port=2
  Memory : Memory  InheritSampleTime=on
  Memory1 : Memory  InheritSampleTime=on
  Memory3 : Memory  InheritSampleTime=on
  P : Product  RndMeth=Zero
  Product : Product  RndMeth=Zero
  Product1 : Product  RndMeth=Zero
  Scope : Scope  NumInputPorts=3
  Scope{1..8} (8 alike) : Scope
  Sign : Signum
  Sign1 : Signum
  Sign2 : Signum
  Sum : Sum  Inputs=|++
  Zero-Order Hold : ZeroOrderHold  SampleTime=0.002
  Zero-Order Hold1 : ZeroOrderHold  SampleTime=0.002
  dV : Sum  Inputs=+-
  dp : Sum  Inputs=+-
  step : Constant  Value=0.5
  signal : Outport
  wires:
  Memory1/1 -> dV/2, Scope/2
  Memory/1 -> dp/2
  Vpv/1 -> Zero-Order Hold1/1, Scope2/1
  dV/1 -> Sign1/1, Scope/3
  step/1 -> Product/2
  Product/1 -> Sum/1, Scope1/1
  Sign/1 -> Product1/1
  Sign1/1 -> Product1/2, Scope7/1
  Product1/1 -> Sign2/1, Scope4/1
  Ipv/1 -> Zero-Order Hold/1, Scope3/1
  Zero-Order Hold1/1 -> P/2, dV/1, Scope/1, Memory1/1
  Zero-Order Hold/1 -> P/1
  P/1 -> Memory/1, dp/1
  dp/1 -> Sign/1, Scope5/1
  Sign2/1 -> Product/1, Scope6/1
  Sum/1 -> Memory3/1, signal/1, Scope8/1
  Memory3/1 -> Sum/2

== system Final_System_Model_V2/Solar Panel + Solar Charge Controller/Solar Charge Controller MPPT it is a device which track a point which has the max power/MPPT /P&O /Subsystem1 ==
  In1 : Inport
  Compare To Zero : simulink/Logic and Bit Operations/Compare To Zero  relop=<=  OutDataTypeStr=boolean
  Repeating Sequence : simulink/Sources/Repeating Sequence  rep_seq_t=[0 0.1e-3]  rep_seq_y=[0 1]
  Subtract : Sum  Inputs=+-
  Out1 : Outport
  wires:
  Subtract/1 -> Compare To Zero/1
  Repeating Sequence/1 -> Subtract/2
  In1/1 -> Subtract/1
  Compare To Zero/1 -> Out1/1

== system Final_System_Model_V2/180KW Fuel Cell Stack/Fuel Cell Model/ From Current Density (A//cm^2) To Overvoltages (V)/Concentration Overvoltage/IF Function/If Action Subsystem ==
  In1 : Inport
  Action Port : ActionPort  ActionType=then
  Math Function1 : Math  Operator=log  OutputSignalType=real  SaturateOnIntegerOverflow=on
  Out1 : Outport
  wires:
  In1/1 -> Math Function1/1
  Math Function1/1 -> Out1/1

== system Final_System_Model_V2/180KW Fuel Cell Stack/Fuel Cell Model/ From Current Density (A//cm^2) To Overvoltages (V)/Concentration Overvoltage/IF Function/If Action Subsystem1 ==
  Action Port : ActionPort  ActionType=else
  Constant1 : Constant  Value=0
  Out1 : Outport
  wires:
  Constant1/1 -> Out1/1

== system Final_System_Model_V2/180KW Fuel Cell Stack/Fuel Cell Model/From Pressures (atm) To Nernest Voltage (V)/From Partial Pressures (atm) To Nernest Voltage (V)/IF Function/If Action Subsystem ==
  In1 : Inport
  Action Port : ActionPort  ActionType=then
  Out1 : Outport
  wires:
  In1/1 -> Out1/1

== system Final_System_Model_V2/180KW Fuel Cell Stack/Fuel Cell Model/From Pressures (atm) To Nernest Voltage (V)/From Partial Pressures (atm) To Nernest Voltage (V)/IF Function/If Action Subsystem1 ==
  In1 : Inport
  Action Port : ActionPort  ActionType=else
  Out1 : Outport
  wires:
  In1/1 -> Out1/1

== system Final_System_Model_V2/Electrolyzer Stack/electrolyser stack/electrolyser cell/Eta_B/segma_B/Beta ==
  In1 : Inport
  In2 : Inport  Port=2
  Add3 : Sum
  Add4 : Sum  Inputs=-+
  Add5 : Sum  Inputs=+-
  Add6 : Sum  Inputs=-+
  Constant3 : Constant
  Constant4 : Constant  Value=4
  Constant5 : Constant  Value=2
  Math Function1 : Math  Operator=square  SaturateOnIntegerOverflow=on
  Product5 : Product  Inputs=***
  Product6 : Product  Inputs=*/
  Product7 : Product  Inputs=*/
  Product8 : Product  Inputs=**
  Sqrt : Sqrt  SaturateOnIntegerOverflow=on
  Out1 : Outport
  wires:
  Math Function1/1 -> Add4/2
  Constant3/1 -> Product6/1, Add5/1, Add3/1
  Add3/1 -> Add6/2, Math Function1/1
  Sqrt/1 -> Add6/1
  Constant4/1 -> Product5/1
  Constant5/1 -> Product8/2
  Add4/1 -> Sqrt/1
  Product6/1 -> Add5/2
  Product5/1 -> Add4/1
  Add6/1 -> Product7/1
  Product8/1 -> Product7/2
  Product7/1 -> Out1/1
  In1/1 -> Product5/2, Add3/2
  In2/1 -> Product6/2
  Add5/1 -> Product8/1, Product5/3

== system Final_System_Model_V2/Electrolyzer Stack/electrolyser stack/electrolyser cell/Eta_B/segma_B/K_a ==
  In1 : Inport
  In2 : Inport  Port=2
  In3 : Inport  Port=3
  Add2 : Sum  Inputs=+-
  Constant : Constant  Value=-523000
  Constant1 : Constant
  Math Function : Math  SaturateOnIntegerOverflow=on
  Product2 : Product  Inputs=*/
  Product3 : Product  Inputs=*/
  Product4 : Product
  Out1 : Outport
  Out2 : Outport  Port=2
  wires:
  Product4/1 -> Math Function/1
  Add2/1 -> Out2/1, Product4/2
  Math Function/1 -> Out1/1
  In3/1 -> Add2/2
  In2/1 -> Product3/2
  Product2/1 -> Product4/1
  Constant1/1 -> Product3/1
  Product3/1 -> Add2/1
  Constant/1 -> Product2/1
  In1/1 -> Product2/2

== system Final_System_Model_V2/Electrolyzer Stack/electrolyser stack/electrolyser cell/Eta_B/segma_B/eta_B ==
  In1 : Inport
  In2 : Inport  Port=2
  Add : Sum
  Product : Product  Inputs=*/
  Out1 : Outport
  wires:
  Product/1 -> Out1/1
  In2/1 -> Add/2
  In1/1 -> Product/1, Add/1
  Add/1 -> Product/2

== system Final_System_Model_V2/Electrolyzer Stack/electrolyser stack/electrolyser cell/Eta_B/segma_B/eta_B0 ==
  In1 : Inport
  In2 : Inport  Port=2
  Add1 : Sum
  Product1 : Product  Inputs=/*
  Out1 : Outport
  wires:
  Add1/1 -> Product1/1
  Product1/1 -> Out1/1
  In1/1 -> Add1/1
  In2/1 -> Product1/2, Add1/2

== system Final_System_Model_V2/Electrolyzer Stack/electrolyser stack/electrolyser cell/eta_a/n_a/i_a0 ==
  In1 : Inport
  In2 : Inport  Port=2
  Divide : Product  Inputs=*/
  E_a : Constant  Value=76
  Exp : Math  SaturateOnIntegerOverflow=on
  Gain : Gain  Gain=-1
  Multiply : Product
  Multiply1 : Product  Inputs=3
  i_a0ref : Constant  Value=5e-12
  lamda_ma : Subsystem
  Out1 : Outport
  wires:
  Gain/1 -> Exp/1
  Exp/1 -> Multiply1/3
  Multiply/1 -> Gain/1
  Divide/1 -> Multiply/1
  i_a0ref/1 -> Multiply1/1
  In2/1 -> Multiply/2
  Multiply1/1 -> Out1/1
  E_a/1 -> Divide/1
  lamda_ma/1(Out1) -> Multiply1/2
  In1/1 -> Divide/2

== system Final_System_Model_V2/Electrolyzer Stack/electrolyser stack/electrolyser cell/eta_c/n_c/i_c0 ==
  In1 : Inport
  In2 : Inport  Port=2
  Divide : Product  Inputs=*/
  E_c : Constant  Value=4.3
  Exp : Math  SaturateOnIntegerOverflow=on
  Gain : Gain  Gain=-1
  Multiply : Product  Inputs=3
  Multiply1 : Product
  i_c0ref : Constant  Value=1e-3
  lamda_mc : Subsystem
  Out1 : Outport
  wires:
  i_c0ref/1 -> Multiply/2
  Multiply/1 -> Out1/1
  Divide/1 -> Multiply1/2
  Multiply1/1 -> Gain/1
  E_c/1 -> Divide/1
  In1/1 -> Divide/2
  lamda_mc/1(Out1) -> Multiply/1
  Exp/1 -> Multiply/3
  Gain/1 -> Exp/1
  In2/1 -> Multiply1/1

== system Final_System_Model_V2/Electrolyzer Stack/electrolyser stack/electrolyser cell/eta_a/n_a/i_a0/lamda_ma ==
  Constant : Constant  Value=6
  Divide : Product  Inputs=*/
  Gain : Gain  Gain=0.75
  Product : Product
  Product1 : Product
  d_ma : Constant  Value=2.9
  m_Ma : Constant  Value=1e-3
  rho_ma : Constant  Value=22.56
  Out1 : Outport
  wires:
  Gain/1 -> Product1/1
  Divide/1 -> Product1/2
  m_Ma/1 -> Gain/1
  d_ma/1 -> Product/2
  rho_ma/1 -> Product/1
  Product/1 -> Divide/2
  Constant/1 -> Divide/1
  Product1/1 -> Out1/1

== system Final_System_Model_V2/Electrolyzer Stack/electrolyser stack/electrolyser cell/eta_c/n_c/i_c0/lamda_mc ==
  Constant : Constant  Value=6
  Divide : Product  Inputs=*/
  Gain : Gain  Gain=0.75
  Multiply : Product
  Multiply1 : Product
  d_mc : Constant  Value=2.7
  m_Mc : Constant  Value=0.3e-3
  rho_mc : Constant  Value=21.45
  Out1 : Outport
  wires:
  Gain/1 -> Multiply1/1
  Divide/1 -> Multiply1/2
  m_Mc/1 -> Gain/1
  Constant/1 -> Divide/1
  d_mc/1 -> Multiply/2
  Multiply/1 -> Divide/2
  Multiply1/1 -> Out1/1
  rho_mc/1 -> Multiply/1

== stateflow chart Final_System_Model_V2/Chart1 ==
  state LOAD [parallel]
    settings: executionOrder=1
    state LOAD_OFF
      entry: load_on=0;
    state LOAD_ON
      entry: load_on=1;
    (default) -> LOAD_OFF
    LOAD_OFF -> LOAD_ON : [load>0]
    LOAD_ON -> LOAD_OFF : [~load>0]
  state Battery [parallel]
    settings: executionOrder=5
    state Battery_Isolated
      entry: pvtobattery=0;
      entry: batterytoload =0;
    state Battery_Charging
      entry: pvtobattery=1;
    state Battery_Discharging
      entry:batterytoload =1;
    (default) -> Battery_Isolated
    Battery_Charging -> Battery_Isolated [order 1] : [(battery_full==1) && (delta<0) ]
    Battery_Isolated -> Battery_Charging [order 2] : [(battery_full==0) && (delta<0) ]
    Battery_Discharging -> Battery_Charging [order 1] : [[delta<0 && battery_full==0]]
    Battery_Charging -> Battery_Discharging [order 2] : [[(delta>0 && delta<72) || (delta>88 && delta<90) || (delta>110 && delta<162) || (delta>198 && delta<215) ]]
    Battery_Isolated -> Battery_Discharging [order 1] : [(delta>0 && delta<72) || (delta>88 && delta<90) || (delta>110 && delta<162) || (delta>198 && delta<215) ]
    Battery_Discharging -> Battery_Isolated [order 2] : [delta<0 || battery_empty==1 || (delta>72 && delta<88) || (delta>90 && delta<110) || (delta>162 && delta<198)]
  state Electrolyser_1 [parallel]
    settings: executionOrder=4
    state Electrolyser_1_OFF
      entry: pvtoelec_1=0;
    state Electrolyser_1_ON
      entry: pvtoelec_1=1;
    (default) -> Electrolyser_1_OFF
    Electrolyser_1_OFF -> Electrolyser_1_ON : [delta<0 && battery_full==1 && tank_full==0]
    Electrolyser_1_ON -> Electrolyser_1_OFF : [delta>=0 || tank_full==1]
  state Electrolyser_2 [parallel]
    settings: executionOrder=6
    state Electrolyser_2_OFF
      entry: pvtoelec_2=0;
    state Electrolyser_2_ON
      entry: pvtoelec_2=1;
    (default) -> Electrolyser_2_OFF
    Electrolyser_2_OFF -> Electrolyser_2_ON : [delta<-260 && battery_full==1 && tank_full==0]
    Electrolyser_2_ON -> Electrolyser_2_OFF : [delta>=0 || tank_full==1]
  state FC_1 [parallel]
    settings: executionOrder=2
    state FC_1_OFF
      entry: fctoload_1=0;
    state FC_1_ON
      entry: fctoload_1=1;
    (default) -> FC_1_OFF
    FC_1_OFF -> FC_1_ON : [(delta>72 && delta<88) || (delta>88 && delta<90) || (delta>162 && delta<198) || (delta>198 && delta<215) ]
    FC_1_ON -> FC_1_OFF : [delta<0]
  state FC_2 [parallel]
    settings: executionOrder=3
    state FC_2_OFF
      entry: fctoload_2=0;
    state FC_2_ON
      entry: fctoload_2=1;
    (default) -> FC_2_OFF
    FC_2_OFF -> FC_2_ON : [(delta>90 && delta<110) || (delta>110 && delta<162) || (delta>198 && delta<215)]
    FC_2_ON -> FC_2_OFF : [delta<0]
  state tank [parallel]
    settings: executionOrder=7
    state tank_Charging
      entry:elect_1totank=1;
      elect_2totank=1;
      resetchargeclock=1;
      exit:resetchargeclock=0;
    state tank_Isolated
      entry: tanktofc_1=0;
      tanktofc_2 =0;
      elect_1totank=0;
      elect_2totank=0;
    state tank_Discharging
      entry:tanktofc_1=1;
      tanktofc_2=1;
      resetdischargeclock=1;
      exit:resetdischargeclock=0;
    (default) -> tank_Isolated
    tank_Isolated -> tank_Charging [order 2] : [(pvtoelec_1==1 || pvtoelec_2==1)]
    tank_Charging -> tank_Isolated [order 2] : [(pvtoelec_1==0 && pvtoelec_2==0)]
    tank_Discharging -> tank_Charging [order 1] : [pvtoelec_1==1||pvtoelec_2==1]
    tank_Charging -> tank_Discharging [order 1] : [pvtoelec_1==0&&pvtoelec_2==0]
    tank_Discharging -> tank_Isolated [order 2] : [fctoload_1==0&&fctoload_2==0]
    tank_Isolated -> tank_Discharging [order 1] : [fctoload_1==1||fctoload_2==1]
  data: battery_full function_input; tank_full function_input; delta2 function_input; fc1toload_on function_output; fc2toload_on function_output; pvtoload_on function_output; batterytoload_on function_output; pvtobattery_on function_output; pvtoelectrolyser_on function_output; load_on output; battery_full1 input; tank_full1 input; delta input; load input; fctoload_1 output; battery_full input; tank_full input; fctoload_2 output; pvtoelec_1 output; pvtobattery output; batterytoload output; battery_empty input; pvtoelec_2 output; tanktofc_1 output; tanktofc_2 output; elect_1totank output; elect_2totank output; resetchargeclock output; resetdischargeclock output
  function [fc1toload_on,fc2toload_on,pvtoload_on,batterytoload_on,pvtobattery_on,pvtoelectrolyser_on] = Operation(battery_full, tank_full, delta2):
    | function [fc1toload_on,fc2toload_on,pvtoload_on,batterytoload_on,pvtobattery_on,pvtoelectrolyser_on] = Operation(battery_full, tank_full, delta2)
    | 
    | aVarTruthTableCondition_1 = false;
    | aVarTruthTableCondition_2 = false;
    | aVarTruthTableCondition_3 = false;
    | aVarTruthTableCondition_4 = false;
    | aVarTruthTableCondition_5 = false;
    | aVarTruthTableCondition_6 = false;
    | aVarTruthTableCondition_7 = false;
    | aVarTruthTableCondition_8 = false;
    | aVarTruthTableCondition_9 = false;
    | aVarTruthTableCondition_10 = false;
    | aVarTruthTableCondition_11 = false;
    | 
    | 
    | % Excess Power
    | 
    | aVarTruthTableCondition_1 = logical(delta<0);
    | 
    | % Battery Full
    | 
    | aVarTruthTableCondition_2 = logical(battery_full==1);
    | 
    | % Tank Full
    | 
    | aVarTruthTableCondition_3 = logical(tank_full==1);
    | 
    | % PV meets Demand
    | 
    | aVarTruthTableCondition_4 = logical(delta==0);
    | 
    | % Shortage1
    | % Battery ON Only
    | 
    | aVarTruthTableCondition_5 = logical(delta<72);
    | 
    | % Shortage2
    | % FC1 Only
    | 
    | aVarTruthTableCondition_6 = logical(delta<88);
    | 
    | % Shortage3
    | % FC1 + Battery
    | 
    | aVarTruthTableCondition_7 = logical(delta<90);
    | 
    | % Shortage4
    | % FC2 Only
    | 
    | aVarTruthTableCondition_8 = logical(delta<110);
    | 
    | % Shortage5
    | %  FC2 + Battery
    | 
    | aVarTruthTableCondition_9 = logical(delta<162);
    | 
    | % Shortage6
    | % FC1 + FC2
    | 
    | aVarTruthTableCondition_10 = logical(delta<198);
    | 
    | % Shortage7
    | % FC1 +FC2 + Battery
    | 
    | aVarTruthTableCondition_11 = logical(delta<214);
    | 
    | if (aVarTruthTableCondition_1 && ~aVarTruthTableCondition_2)
    |     A1();
    | elseif (aVarTruthTableCondition_1 && aVarTruthTableCondition_2 && ~aVarTruthTableCondition_3)
    |     A2();
    | elseif (aVarTruthTableCondition_4)
    |     A3();
    | elseif (~aVarTruthTableCondition_4 && aVarTruthTableCondition_5)
    |     A4();
    | elseif (~aVarTruthTableCondition_5 && aVarTruthTableCondition_6)
    |     A5();
    | elseif (~aVarTruthTableCondition_6 && aVarTruthTableCondition_7)
    |     A6();
    | elseif (~aVarTruthTableCondition_7 && aVarTruthTableCondition_8)
    |     A7();
    | elseif (~aVarTruthTableCondition_8 && aVarTruthTableCondition_9)
    |     A8();
    | elseif (~aVarTruthTableCondition_9 && aVarTruthTableCondition_10)
    |     A9();
    | elseif (~aVarTruthTableCondition_10 && aVarTruthTableCondition_11)
    |     A10();
    | elseif (aVarTruthTableCondition_1 && aVarTruthTableCondition_2 && aVarTruthTableCondition_3)
    |     A11();
    | else % Default
    |     DA();
    | end
    | 
    | function A1()
    | 
    | % Excess Power ِAND Battery Empty
    | 
    | fc1toload_on=0;
    | fc2toload_on=0;
    | pvtoload_on=1;
    | batterytoload_on=0;
    | pvtobattery_on=1;
    | pvtoelectrolyser_on=0;
    | 
    | function A2()
    | 
    | % Excess power AND Battery Full AND Tank Empty
    | 
    | fc1toload_on=0;
    | fc2toload_on=0;
    | pvtoload_on=1;
    | batterytoload_on=0;
    | pvtobattery_on=0;
    | pvtoelectrolyser_on=1;
    | 
    | function A3()
    | 
    | % PV meets Demand
    | 
    | fc1toload_on=0;
    | fc2toload_on=0;
    | pvtoload_on=1;
    | batterytoload_on=0;
    | pvtobattery_on=0;
    | pvtoelectrolyser_on=0;
    | 
    | function A4()
    | 
    | % Shortage1
    | % Battery ON Only
    | 
    | fc1toload_on=0;
    | fc2toload_on=0;
    | pvtoload_on=1;
    | batterytoload_on=1;
    | pvtobattery_on=0;
    | pvtoelectrolyser_on=0;
    | 
    | function A5()
    | 
    | % Shortage2
    | % FC1 Only
    | 
    | fc1toload_on=1;
    | fc2toload_on=0;
    | pvtoload_on=1;
    | batterytoload_on=0;
    | pvtobattery_on=0;
    | pvtoelectrolyser_on=0;
    | 
    | function A6()
    | 
    | % Shortage3
    | % FC1 + Battery
    | 
    | fc1toload_on=1;
    | fc2toload_on=0;
    | pvtoload_on=1;
    | batterytoload_on=1;
    | pvtobattery_on=0;
    | pvtoelectrolyser_on=0;
    | 
    | function A7()
    | 
    | % Shortage4
    | % FC2 Only
    | 
    | fc1toload_on=0;
    | fc2toload_on=1;
    | pvtoload_on=1;
    | batterytoload_on=0;
    | pvtobattery_on=0;
    | pvtoelectrolyser_on=0;
    | 
    | function A8()
    | 
    | % Shortage5
    | %  FC2 + Battery
    | 
    | fc1toload_on=0;
    | fc2toload_on=1;
    | pvtoload_on=1;
    | batterytoload_on=1;
    | pvtobattery_on=0;
    | pvtoelectrolyser_on=0;
    | 
    | function A9()
    | 
    | % Shortage6
    | % FC1 + FC2
    | 
    | fc1toload_on=1;
    | fc2toload_on=1;
    | pvtoload_on=1;
    | batterytoload_on=0;
    | pvtobattery_on=0;
    | pvtoelectrolyser_on=0;
    | 
    | function A10()
    | 
    | % Shortage7
    | % FC1 +FC2 + Battery
    | 
    | fc1toload_on=1;
    | fc2toload_on=1;
    | pvtoload_on=1;
    | batterytoload_on=1;
    | pvtobattery_on=0;
    | pvtoelectrolyser_on=0;
    | 
    | function DA()
    | 
    | % Default
    | 
    | fc1toload_on=0;
    | fc2toload_on=0;
    | pvtoload_on=0;
    | batterytoload_on=0;
    | pvtobattery_on=0;
    | pvtoelectrolyser_on=0;
    | 
    | function A11()
    | 
    | % Excess Power AND Battery Full AND Tank Full
    | 
    | fc1toload_on=0;
    | fc2toload_on=0;
    | pvtoload_on=1;
    | batterytoload_on=0;
    | pvtobattery_on=0;
    | pvtoelectrolyser_on=0;

== stateflow chart Final_System_Model_V2/OLD Version Models/Chart ==
  state pvLogic [parallel]
    settings: executionOrder=1
    state pvOFF
      entry: pv_on=0;
      during: fc_mode=1;
    state pvON
      entry: pv_on=1;
    (default) -> pvOFF
    pvOFF -> pvON : [isActive(V_pv)]
        | {fc_mode=0;}
    pvON -> pvOFF : [~isActive(V_pv)]
  state fcLogic [parallel] [commented out]
    state fcON [commented out]
      entry: Vfc=1
    state fcOFF [commented out]
      entry: Vfc=0;
    (default) -> fcOFF [commented out]
    fcOFF -> fcON [commented out] : [fc_mode==1 && isActive(V_fc)]
    fcON -> fcOFF [commented out] : [fc_mode==0 || ~isActive(V_fc)]
  state alarmLogic [parallel] [commented out]
    state alarmOFF [commented out]
      entry: alarm=0;
    state alarmON [commented out]
      entry:alarm=1;
    (default) -> alarmOFF [commented out]
    alarmOFF -> alarmON [commented out] : [pv_on==0 && Vfc==0]
    alarmON -> alarmOFF [commented out] : [pv_on || Vfc]
  state status = isActive(V) [function] [commented out]
    (default) -> (junction 35) [commented out]
    (junction 35) -> (junction 36) [commented out] : [V>=60]
    (junction 35) -> (junction 37) [commented out] : {status=0;}
    (junction 36) -> (junction 38) [commented out] : {status=1;}
    (junction 38) -> (junction 37) [commented out]
    (junction 37) -> (junction 39) [commented out]
  data: V function_input; status function_output; switch_on input; pv_on output; V_pv input; Vfc output; fc_mode local; alarm output; V_fc input
  function operation:
    | function operation

== matlab function Final_System_Model_V2/OLD Version Models/ClimateController1 ==
  data: delta input; battery_full input; tank_full input; fc1toload_on output; fc2toload_on output; pvtoload_on output; batterytoload_on output; pvtobattery_on output; pvtoelectrolyser_on output
function [fc1toload_on, fc2toload_on, pvtoload_on, batterytoload_on, pvtobattery_on, pvtoelectrolyser_on] = fcn(delta, battery_full, tank_full)

aVarTruthTableCondition_1 = false;
aVarTruthTableCondition_2 = false;
aVarTruthTableCondition_3 = false;
aVarTruthTableCondition_4 = false;
aVarTruthTableCondition_5 = false;
aVarTruthTableCondition_6 = false;
aVarTruthTableCondition_7 = false;
aVarTruthTableCondition_8 = false;
aVarTruthTableCondition_9 = false;
aVarTruthTableCondition_10 = false;
aVarTruthTableCondition_11 = false;


% Excess Power

aVarTruthTableCondition_1 = logical(delta<0);

% Battery Full

aVarTruthTableCondition_2 = logical(battery_full==1);

% Tank Full

aVarTruthTableCondition_3 = logical(tank_full==1);

% PV meets Demand

aVarTruthTableCondition_4 = logical(delta==0);

% Shortage1
% Battery ON Only

aVarTruthTableCondition_5 = logical(delta<72);

% Shortage2
% FC1 Only

aVarTruthTableCondition_6 = logical(delta<88);

% Shortage3
% FC1 + Battery

aVarTruthTableCondition_7 = logical(delta<90);

% Shortage4
% FC2 Only

aVarTruthTableCondition_8 = logical(delta<110);

% Shortage5
%  FC2 + Battery

aVarTruthTableCondition_9 = logical(delta<162);

% Shortage5
%  FC2 + Battery

aVarTruthTableCondition_10 = logical(delta<198);

% Shortage7
% FC1 +FC2 + Battery

aVarTruthTableCondition_11 = logical(delta<215);

if (aVarTruthTableCondition_1 && ~aVarTruthTableCondition_2)
    A1();
elseif (aVarTruthTableCondition_1 && aVarTruthTableCondition_2 && ~aVarTruthTableCondition_3)
    A2();
elseif (aVarTruthTableCondition_4)
    A3();
elseif (~aVarTruthTableCondition_1 && ~aVarTruthTableCondition_4 && aVarTruthTableCondition_5)
    A4();
elseif (~aVarTruthTableCondition_5 && aVarTruthTableCondition_6)
    A5();
elseif (~aVarTruthTableCondition_6 && aVarTruthTableCondition_7)
    A6();
elseif (~aVarTruthTableCondition_7 && aVarTruthTableCondition_8)
    A7();
elseif (~aVarTruthTableCondition_8 && aVarTruthTableCondition_9)
    A8();
elseif (~aVarTruthTableCondition_9 && aVarTruthTableCondition_10)
    A9();
elseif (~aVarTruthTableCondition_10 && aVarTruthTableCondition_11)
    A10();
elseif (aVarTruthTableCondition_1 && aVarTruthTableCondition_2 && aVarTruthTableCondition_3)
    A11();
else % Default
    DA();
end

function A1()

% Excess Power ِAND Battery Empty

fc1toload_on=0;
fc2toload_on=0;
pvtoload_on=1;
batterytoload_on=0;
pvtobattery_on=1;
pvtoelectrolyser_on=0;

function A2()

% Excess power AND Battery Full AND Tank Empty

fc1toload_on=0;
fc2toload_on=0;
pvtoload_on=1;
batterytoload_on=0;
pvtobattery_on=0;
pvtoelectrolyser_on=1;

function A3()

% PV meets Demand

fc1toload_on=0;
fc2toload_on=0;
pvtoload_on=1;
batterytoload_on=0;
pvtobattery_on=0;
pvtoelectrolyser_on=0;

function A4()

% Shortage1
% Battery ON Only

fc1toload_on=0;
fc2toload_on=0;
pvtoload_on=1;
batterytoload_on=1;
pvtobattery_on=0;
pvtoelectrolyser_on=0;

function A5()

% Shortage2
% FC1 Only

fc1toload_on=1;
fc2toload_on=0;
pvtoload_on=1;
batterytoload_on=0;
pvtobattery_on=0;
pvtoelectrolyser_on=0;

function A6()

% Shortage3
% FC1 + Battery

fc1toload_on=1;
fc2toload_on=0;
pvtoload_on=1;
batterytoload_on=1;
pvtobattery_on=0;
pvtoelectrolyser_on=0;

function A7()

% Shortage4
% FC2 Only

fc1toload_on=0;
fc2toload_on=1;
pvtoload_on=1;
batterytoload_on=0;
pvtobattery_on=0;
pvtoelectrolyser_on=0;

function A8()

% Shortage5
%  FC2 + Battery

fc1toload_on=0;
fc2toload_on=1;
pvtoload_on=1;
batterytoload_on=1;
pvtobattery_on=0;
pvtoelectrolyser_on=0;

function A9()

% Shortage6
% FC1 + FC2

fc1toload_on=1;
fc2toload_on=1;
pvtoload_on=1;
batterytoload_on=0;
pvtobattery_on=0;
pvtoelectrolyser_on=0;

function A10()

% Shortage7
% FC1 +FC2 + Battery

fc1toload_on=1;
fc2toload_on=1;
pvtoload_on=1;
batterytoload_on=1;
pvtobattery_on=0;
pvtoelectrolyser_on=0;

function DA()

% Default

fc1toload_on=0;
fc2toload_on=0;
pvtoload_on=0;
batterytoload_on=0;
pvtobattery_on=0;
pvtoelectrolyser_on=0;

function A11()

% Excess Power AND Battery Full AND Tank Full

fc1toload_on=0;
fc2toload_on=0;
pvtoload_on=1;
batterytoload_on=0;
pvtobattery_on=0;
pvtoelectrolyser_on=0;
